simulink model "mysim"  (R2014a)
settings: Solver=ode45  StartTime=0.0  StopTime=10.0  RelTol=1e-3
libraries: vrlib x3, slrtlib x2
settings Model: SimulationMode=external  Creator=Bignell  LastModifiedBy=Bignell

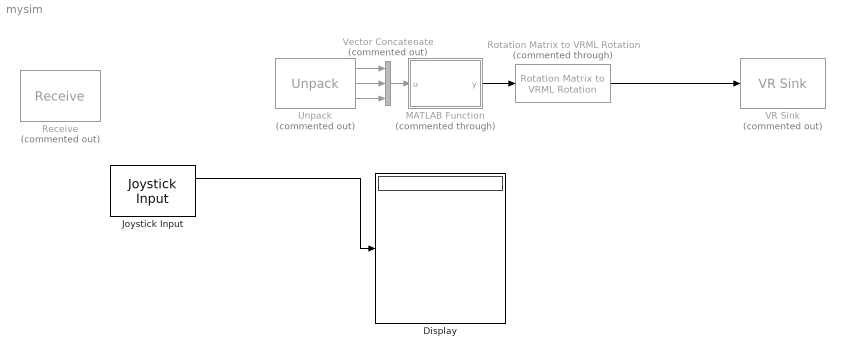
== system mysim ==
  Display : Display
  Joystick Input : vrlib/Joystick Input  joyid=1  adjustports=on  forcefeed=off
  MATLAB Function : MATLAB Function  Commented=through  TreatAsAtomicUnit=on
  "Receive " : slrtlib/UDP/Receive   Commented=on  ipAddress=0.0.0.0  ipPort=25000  width=1  vblLen=off  sampletime=0.01
  Rotation Matrix to VRML Rotation : vrlib/Utilities/Rotation Matrix to VRML Rotation  Commented=through  maxzero=1e-12
  "Unpack " : slrtlib/UDP/Unpack   Commented=on  dimensions={[1],[2],[3]}  datatypes={'double','double','double'}  byteAlign=1
  VR Sink : vrlib/VR Sink  Commented=on  InstantiateOnLoad=on  SampleTime=0.1  ViewEnable=on  RemoteChange=off  RemoteView=off  FieldsWritten=BaseRotation.rotation.4.1.1.double  WorldFileName=world.wrl  AutoView=off  VideoDimensions=[]  AllowVariableSize=off
  Vector Concatenate : Concatenate  Commented=on  NumInputs=3
  wires:
  "Unpack "/1 -> Vector Concatenate/1
  "Unpack "/2 -> Vector Concatenate/2
  "Unpack "/3 -> Vector Concatenate/3
  Vector Concatenate/1 -> MATLAB Function/1(u)
  MATLAB Function/1(y) -> Rotation Matrix to VRML Rotation/1
  Rotation Matrix to VRML Rotation/1 -> VR Sink/1
  Joystick Input/1 -> Display/1

== matlab function mysim/MATLAB Function ==
  data: u input; y output
function y = fcn(u)
%#codegen


    phi = u(1);  %rotation about x-axis, gamma 
    th  = u(2);  % rotation about y-axis, beta
    psi = u(3);  % rotation about z-axis, alpha
    
    %STEP 2: Elements r_ij of BP_R = Rzyx
    % Calculate the required sines and cosines
    cphi = cos(phi); 
    sphi = sin(phi);
    cth  = cos(th);  
    sth  = sin(th);
    cpsi = cos(psi); 
    spsi = sin(psi);
    
    % Calculate the rotation matrix
    Rzyx = [cpsi*cth      cpsi*sth*sphi - spsi*cphi     cpsi*sth*cphi + spsi*sphi;
            spsi*cth      spsi*sth*sphi + cpsi*cphi     spsi*sth*cphi - cpsi*sphi;
            -sth          cth*sphi                      cth*cphi];
        
    y = Rzyx;


y = u;
